simulink model "simulink_scenario_reader"  (R2022a)
settings: Solver=FixedStepAuto  StartTime=0.0  StopTime=10.0  RelTol=1e-3
model workspace (MAT data in the model file):
  firstWarning = 0
  originalScenarioChecksum = 'E48F73370D4002DBAA47AD0521C44C41'
undefined symbols (not defined in the file or in its folder): driving
libraries: drivingscenarioandsensors x6, sim3dautolib x2, trackingutilitieslib x1, sim3dlib x1
settings Model: Creator=bighsiao  LastModifiedBy=bighsiao

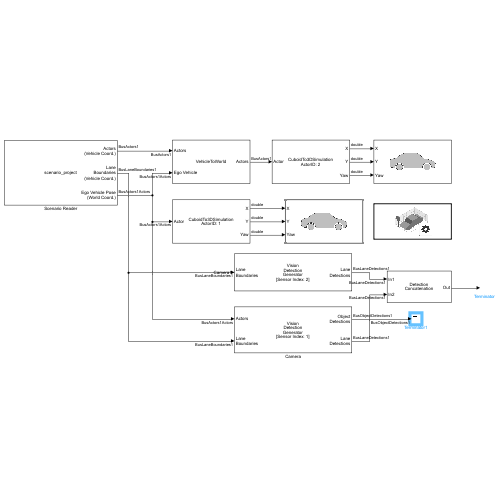
[thumbnail: Simulink's stored preview of the top-level diagram]
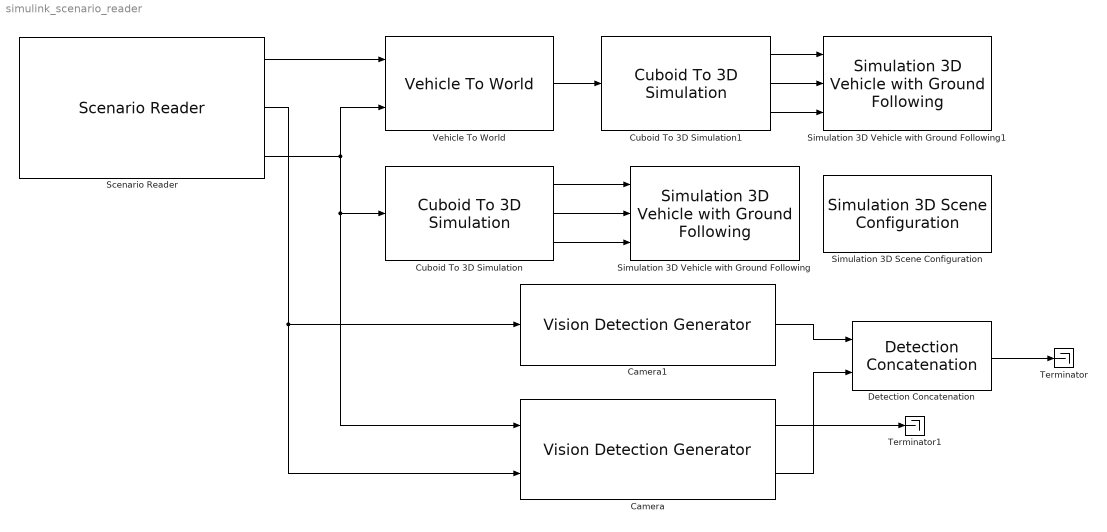
== system simulink_scenario_reader ==
  Camera : drivingscenarioandsensors/Vision Detection Generator  SensorIndex=1  DetectorOutput=Lanes and objects  UpdateInterval=0.1  LaneUpdateInterval=0.1  SensorLocation=[1.9 0]  Height=1.1  Yaw=0  Pitch=1  Roll=0  BusNameSource=Auto  BusName=BusObjectDetections  BusName2Source=Auto  BusName2=BusLaneDetections  MaxNumDetectionsSource=Property  MaxNumDetections=50  MaxNumLanesSource=Property  MaxNumLanes=30  DetectionCoordinates=Ego Cartesian  SimulateUsing=Interpreted execution  MaxRange=100  BoundingBoxAccuracy=5  ProcessNoiseIntensity=5  MaxSpeed=100  MaxAllowedOcclusion=0.5  MinObjectImageSize=[15 15]  DetectionProbability=0.9  FalsePositivesPerImage=0.1  MinLaneImageSize=[20 3]  LaneBoundaryAccuracy=3  HasNoise=on  InitialSeedSource=Repeatable  InitialSeed=0  UsedSeed=0  ActorProfilesSource=From Scenario Reader block  ActorProfilesParameters=driving.internal.ActorProfilesParameters  ActorProfilesExpression=[struct('ActorID',1,'ClassID',1,'Length',4.7,'Width',1.8,'Height',1.4,'OriginOffset',[-1.35 0 0],'MeshVertices',[3.7 0.9 0.857439446366782;3.7 -0.9 0.857439446366782;3.7 -0.9 0.314878892733564;3.7 0.9 0.314878892733564;3.7 0.9 0.857439446366782;2.525 0.9 0.993079584775086;2.525 -0.9 0.993079584775086;3.7 -0.9 0.857439446366782;1.82 0.72 1.4;0.41 0.72 1.4;0.41 -0.72 1.4;1.82 -0.72 1.4;-0.295 0.9 0.993079584775086;-1 0.9 0.857439446366782;-1 -0.9 0.857439446366782;-0.295 -0.9 0.993079584775086;3.7 0.9 0.857439446366782;3.7 0.9 0.314878892733564;2.525 0.9 0.314878892733564;2.525 0.9 0.993079584775086;2.525 0.9 0.993079584775086;2.525 0.9 0.314878892733564;-0.295 0.9 0.314878892733564;-0.295 0.9 0.993079584775086;-0.295 0.9 0.993079584775086;-0.295 0.9 0.314878892733564;-1 0.9 0.355570934256055;-1 0.9 0.857439446366782;2.525 0.9 0.993079584775086;-0.295 0.9 0.993079584775086;0.41 0.72 1.4;1.82 0.72 1.4;3.7 -0.9 0.857439446366782;3.7 -0.9 0.314878892733564;2.525 -0.9 0.314878892733564;2.525 -0.9 0.993079584775086;2.525 -0.9 0.993079584775086;2.525 -0.9 0.314878892733564;-0.295 -0.9 0.314878892733564;-0.295 -0.9 0.993079584775086;-0.295 -0.9 0.993079584775086;-0.295 -0.9 0.314878892733564;-1 -0.9 0.355570934256055;-1 -0.9 0.857439446366782;2.525 -0.9 0.993079584775086;-0.295 -0.9 0.993079584775086;0.41 -0.72 1.4;1.82 -0.72 1.4;-0.295 0.9 0.993079584775086;-0.295 -0.9 0.993079584775086;0.41 -0.72 1.4;0.41 0.72 1.4;2.525 -0.9 0.993079584775086;1.82 -0.72 1.4;1.82 0.72 1.4;2.525 0.9 0.993079584775086;-1 0.9 0.857439446366782;-1 0.9 0.355570934256055;-1 -0.9 0.355570934256055;-1 -0.9 0.857439446366782;3.7 0.9 0.314878892733564;3.7 -0.9 0.314878892733564;-0.295 -0.9 0.314878892733564;-0.295 0.9 0.314878892733564;-0.295 0.9 0.314878892733564;-1 0.9 0.355570934256055;-1 -0.9 0.355570934256055;-0.295 -0.9 0.314878892733564;0 -0.63 0;0 -0.87 0;0.191030206995054 -0.63 0.0601365173421445;0.191030206995054 -0.87 0.0601365173421445;0.309093367795925 -0.63 0.217575963708927;0.309093367795925 -0.87 0.217575963708927;0.309093367795925 -0.63 0.412181821758201;0.309093367795925 -0.87 0.412181821758201;0.191030206995054 -0.63 0.569621268124983;0.191030206995054 -0.87 0.569621268124983;0 -0.63 0.629757785467128;0 -0.87 0.629757785467128;-0.191030206995054 -0.63 0.569621268124983;-0.191030206995054 -0.87 0.569621268124983;-0.309093367795925 -0.63 0.412181821758201;-0.309093367795925 -0.87 0.412181821758201;-0.309093367795925 -0.63 0.217575963708927;-0.309093367795925 -0.87 0.217575963708927;-0.191030206995054 -0.63 0.0601365173421445;-0.191030206995054 -0.87 0.0601365173421445;0 -0.63 0;0 -0.87 0;0 -0.63 0;0.191030206995054 -0.63 0.0601365173421445;0.309093367795925 -0.63 0.217575963708927;0.309093367795925 -0.63 0.412181821758201;0.191030206995054 -0.63 0.569621268124983;0 -0.63 0.629757785467128;-0.191030206995054 -0.63 0.569621268124983;-0.309093367795925 -0.63 0.412181821758201;-0.309093367795925 -0.63 0.217575963708927;-0.191030206995054 -0.63 0.0601365173421445;0 -0.87 0;0.191030206995054 -0.87 0.0601365173421445;0.309093367795925 -0.87 0.217575963708927;0.309093367795925 -0.87 0.412181821758201;0.191030206995054 -0.87 0.569621268124983;0 -0.87 0.629757785467128;-0.191030206995054 -0.87 0.569621268124983;-0.309093367795925 -0.87 0.412181821758201;-0.309093367795925 -0.87 0.217575963708927;-0.191030206995054 -0.87 0.0601365173421445;0 0.87 0;0 0.63 0;0.191030206995054 0.87 0.0601365173421445;0.191030206995054 0.63 0.0601365173421445;0.309093367795925 0.87 0.217575963708927;0.309093367795925 0.63 0.217575963708927;0.309093367795925 0.87 0.412181821758201;0.309093367795925 0.63 0.412181821758201;0.191030206995054 0.87 0.569621268124983;0.191030206995054 0.63 0.569621268124983;0 0.87 0.629757785467128;0 0.63 0.629757785467128;-0.191030206995054 0.87 0.569621268124983;-0.191030206995054 0.63 0.569621268124983;-0.309093367795925 0.87 0.412181821758201;-0.309093367795925 0.63 0.412181821758201;-0.309093367795925 0.87 0.217575963708927;-0.309093367795925 0.63 0.217575963708927;-0.191030206995054 0.87 0.0601365173421445;-0.191030206995054 0.63 0.0601365173421445;0 ...(+3718 chars)],'MeshFaces',[1 2 3;3 4 1;5 6 7;7 8 5;9 10 11;11 12 9;13 14 15;15 16 13;17 18 19;19 20 17;21 22 23;23 24 21;25 26 27;27 28 25;29 30 31;31 32 29;33 34 35;35 36 33;37 38 39;39 40 37;41 42 43;43 44 41;45 46 47;47 48 45;49 50 51;51 52 49;53 54 55;55 56 53;57 58 59;59 60 57;61 62 63;63 64 61;65 66 67;67 68 65;69 71 72;72 70 69;71 73 74;74 72 71;73 75 76;76 74 73;75 77 78;78 76 75;77 79 80;80 78 77;79 81 82;82 80 79;81 83 84;84 82 81;83 85 86;86 84 83;85 87 88;88 86 85;87 89 90;90 88 87;91 92 93;91 93 94;91 94 95;91 95 96;91 96 97;91 97 98;91 98 99;91 99 100;101 102 103;101 103 104;101 104 105;101 105 106;101 106 107;101 107 108;101 108 109;101 109 110;111 113 114;114 112 111;113 115 116;116 114 113;115 117 118;118 116 115;117 119 120;120 118 117;119 121 122;122 120 119;121 123 124;124 122 121;123 125 126;126 124 123;125 127 128;128 126 125;127 129 130;130 128 127;129 131 132;132 130 129;133 134 135;133 135 136;133 136 137;133 137 138;133 138 139;133 139 140;133 140 141;133 141 142;143 144 145;143 145 146;143 146 147;143 147 148;143 148 149;143 149 150;143 150 151;143 151 152;153 155 156;156 154 153;155 157 158;158 156 155;157 159 160;160 158 157;159 161 162;162 160 159;161 163 164;164 162 161;163 165 166;166 164 163;165 167 168;168 166 165;167 169 170;170 168 167;169 171 172;172 170 169;171 173 174;174 172 171;175 176 177;175 177 178;175 178 179;175 179 180;175 180 181;175 181 182;175 182 183;175 183 184;185 186 187;185 187 188;185 188 189;185 189 190;185 190 191;185 191 192;185 192 193;185 193 194;195 197 198;198 196 195;197 199 200;200 198 197;199 201 202;202 200 199;201 203 204;204 202 201;203 205 206;206 204 203;205 207 208;208 206 205;207 209 210;210 208 207;209 211 212;212 210 209;211 213 214;214 212 211;213 215 216;216 214 213;217 218 219;217 219 220;217 220 221;217 221 222;217 222 223;217 223 224;217 224 225;217 225 226;227 228 229;227 229 230;227 230 231;227 231 232;227 232 233;227 233 234;227 234 235;227 235 236],'RCSPattern',[10 10;10 10],'RCSAzimuthAngles',[-180 180],'RCSElevationAngles',[-90 90]); struct('ActorID',2,'ClassID',2,'Length',8.2,'Width',2.5,'Height',3.5,'OriginOffset',[-3.1 0 0],'MeshVertices',[7.2 1.25 1.30597014925373;7.2 -1.25 1.30597014925373;7.2 -1.25 0.574626865671641;7.2 1.25 0.574626865671641;7.2 1.25 1.30597014925373;5.765 1.25 1.67164179104478;5.765 -1.25 1.67164179104478;7.2 -1.25 1.30597014925373;4.945 1 2.58582089552239;4.002 1 2.58582089552239;4.002 -1 2.58582089552239;4.945 -1 2.58582089552239;4.002 1 2.58582089552239;4.002 1.25 1.67164179104478;4.002 -1.25 1.67164179104478;4.002 -1 2.58582089552239;4.002 1.25 1.67164179104478;4.002 1.25 0.574626865671641;4.002 -1.25 0.574626865671641;4.002 -1.25 1.67164179104478;3.92 1.25 3.5;-1 1.25 3.5;-1 -1.25 3.5;3.92 -1.25 3.5;3.92 -1.25 3.5;3.92 -1.25 0.574626865671641;3.92 1.25 0.574626865671641;3.92 1.25 3.5;-1 1.25 3.5;-1 1.25 0.574626865671641;3.92 1.25 0.574626865671641;3.92 1.25 3.5;-1 -1.25 3.5;-1 -1.25 0.574626865671641;3.92 -1.25 0.574626865671641;3.92 -1.25 3.5;5.765 1.25 1.67164179104478;5.355 1.25 1.67164179104478;4.74 1 2.58582089552239;4.945 1 2.58582089552239;7.2 1.25 1.30597014925373;7.2 1.25 0.574626865671641;5.765 1.25 0.574626865671641;5.765 1.25 1.67164179104478;5.765 1.25 1.67164179104478;5.765 1.25 0.574626865671641;4.002 1.25 0.574626865671641;4.002 1.25 1.67164179104478;4.33 1.25 1.67164179104478;4.002 1.25 1.67164179104478;4.002 1 2.58582089552239;4.33 1 2.58582089552239;5.765 -1.25 1.67164179104478;5.355 -1.25 1.67164179104478;4.74 -1 2.58582089552239;4.945 -1 2.58582089552239;7.2 -1.25 1.30597014925373;7.2 -1.25 0.574626865671641;5.765 -1.25 0.574626865671641;5.765 -1.25 1.67164179104478;5.765 -1.25 1.67164179104478;5.765 -1.25 0.574626865671641;4.002 -1.25 0.574626865671641;4.002 -1.25 1.67164179104478;4.33 -1.25 1.67164179104478;4.002 -1.25 1.67164179104478;4.002 -1 2.58582089552239;4.33 -1 2.58582089552239;-1 1.25 3.5;-1 1.25 0.574626865671641;-1 -1.25 0.574626865671641;-1 -1.25 3.5;7.2 1.25 0.574626865671641;7.2 -1.25 0.574626865671641;-1 -1.25 0.574626865671641;-1 1.25 0.574626865671641;0 -0.915 -2.22044604925031e-16;0 -1.185 -2.22044604925031e-16;0.293892626146237 -0.915 0.0997672417444302;0.293892626146237 -1.185 0.0997672417444302;0.475528258147577 -0.915 0.360961271595177;0.475528258147577 -1.185 0.360961271595177;0.475528258147577 -0.915 0.683814847807808;0.475528258147577 -1.185 0.683814847807808;0.293892626146237 -0.915 0.945008877658554;0.293892626146237 -1.185 0.945008877658554;0 -0.915 1.04477611940298;0 -1.185 1.04477611940298;-0.293892626146237 -0.915 0.945008877658554;-0.293892626146237 -1.185 0.945008877658554;-0.475528258147577 -0.915 0.683814847807808;-0.475528258147577 -1.185 0.683814847807808;-0.475528258147577 -0.915 0.360961271595177;-0.475528258147577 -1.185 0.360961271595177;-0.293892626146237 -0.915 0.0997672417444302;-0.293892626146237 -1.185 0.0997672417444302;0 -0.915 -2.22044604925031e-16;0 -1.185 -2.22044604925031e-16;0 -0.915 -2.22044604925031e-16;0.293892626146237 -0.915 0.0997672417444302;0.475528258147577 -0.915 0.360961271595177;0.475528258147577 -0.915 0.683814847807808;0.293892626146237 -0.915 0.945008877658554;0 -0.915 1.04477611940298;-0.293892626146237 -0.915 0.945008877658554;-0.475528258147577 -0.915 0.683814847807808;-0.475528258147577 -0.915 0.360961271595177;-0.293892626146237 -0.915 0.0997672417444302;0 -1.185 -2.22044604925031e-16;0.293892626146237 -1.185 0.0997672417444302;0.475528258147577 -1.185 0.360961271595177;0.475528258147577 -1.185 0.683814847807808;0.293892626146237 -1.185 0.945008877658554;0 -1.185 1.04477611940298;-0.293892626146237 -1.185 0.945008877658554;-0.475528258147577 -1.185 0.683814847807808;-0.475528258147577 -1.185 0.360961271595177;-0.293892626146237 -1.185 0.0997672417444302;0 1.185 -2.22044604925031e-16;0 0.915 -2.22044604925031e-16;0.293892626146237 1.185 0.0997672417444302;0.293892626146237 0.915 0.0997672417444302;0.475528258147577 1.185 0.360961271595177;0.475528258147577 0.915 0.360961271595177;0.475528258147577 1.185 0.683814847807808;0.475528258147577 0.915 0.683814847807808;0.293892626146237 1.185 0.945008877658554;0.293892626146237 0.915 ...(+7888 chars)],'MeshFaces',[1 2 3;3 4 1;5 6 7;7 8 5;9 10 11;11 12 9;13 14 15;15 16 13;17 18 19;19 20 17;21 22 23;23 24 21;25 26 27;27 28 25;29 30 31;31 32 29;33 34 35;35 36 33;37 38 39;39 40 37;41 42 43;43 44 41;45 46 47;47 48 45;49 50 51;51 52 49;53 54 55;55 56 53;57 58 59;59 60 57;61 62 63;63 64 61;65 66 67;67 68 65;69 70 71;71 72 69;73 74 75;75 76 73;77 79 80;80 78 77;79 81 82;82 80 79;81 83 84;84 82 81;83 85 86;86 84 83;85 87 88;88 86 85;87 89 90;90 88 87;89 91 92;92 90 89;91 93 94;94 92 91;93 95 96;96 94 93;95 97 98;98 96 95;99 100 101;99 101 102;99 102 103;99 103 104;99 104 105;99 105 106;99 106 107;99 107 108;109 110 111;109 111 112;109 112 113;109 113 114;109 114 115;109 115 116;109 116 117;109 117 118;119 121 122;122 120 119;121 123 124;124 122 121;123 125 126;126 124 123;125 127 128;128 126 125;127 129 130;130 128 127;129 131 132;132 130 129;131 133 134;134 132 131;133 135 136;136 134 133;135 137 138;138 136 135;137 139 140;140 138 137;141 142 143;141 143 144;141 144 145;141 145 146;141 146 147;141 147 148;141 148 149;141 149 150;151 152 153;151 153 154;151 154 155;151 155 156;151 156 157;151 157 158;151 158 159;151 159 160;161 163 164;164 162 161;163 165 166;166 164 163;165 167 168;168 166 165;167 169 170;170 168 167;169 171 172;172 170 169;171 173 174;174 172 171;173 175 176;176 174 173;175 177 178;178 176 175;177 179 180;180 178 177;179 181 182;182 180 179;183 184 185;183 185 186;183 186 187;183 187 188;183 188 189;183 189 190;183 190 191;183 191 192;193 194 195;193 195 196;193 196 197;193 197 198;193 198 199;193 199 200;193 200 201;193 201 202;203 205 206;206 204 203;205 207 208;208 206 205;207 209 210;210 208 207;209 211 212;212 210 209;211 213 214;214 212 211;213 215 216;216 214 213;215 217 218;218 216 215;217 219 220;220 218 217;219 221 222;222 220 219;221 223 224;224 222 221;225 226 227;225 227 228;225 228 229;225 229 230;225 230 231;225 231 232;225 232 233;225 233 234;235 236 237;235 237 238;235 238 239;235 239 240;235 240 241;235 241 242;235 242 243;235 243 244;245 247 248;248 246 245;247 249 250;250 248 247;249 251 252;252 250 249;251 253 254;254 252 251;253 255 256;256 254 253;255 257 258;258 256 255;257 259 260;260 258 257;259 261 262;262 260 259;261 263 264;264 262 261;263 265 266;266 264 263;267 268 269;267 269 270;267 270 271;267 271 272;267 272 273;267 273 274;267 274 275;267 275 276;277 278 279;277 279 280;277 280 281;277 281 282;277 282 283;277 283 284;277 284 285;277 285 286;287 289 290;290 288 287;289 291 292;292 290 289;291 293 294;294 292 291;293 295 296;296 294 293;295 297 298;298 296 295;297 299 300;300 298 297;299 301 302;302 300 299;301 303 304;304 302 301;303 305 306;306 304 303;305 307 308;308 306 305;309 310 311;309 311 312;309 312 313;309 313 314;309 314 315;309 315 316;309 316 317;309 317 318;319 320 321;319 321 322;319 322 323;319 323 324;319 324 325;319 325 326;319 326 327;319 327 328],'RCSPattern',[10 10;10 10],'RCSAzimuthAngles',[-180 180],'RCSElevationAngles',[-90 90])]  Intrinsics=driving.internal.cameraIntrinsics('FocalLength',[500 1814.81],'PrincipalPoint',[320 240],'ImageSize',[720 480],'RadialDistortion',[0 0],'TangentialDistortion',[0 0],'Skew',0)
  Camera1 : drivingscenarioandsensors/Vision Detection Generator  SensorIndex=2  DetectorOutput=Lanes only  UpdateInterval=0.1  LaneUpdateInterval=0.1  SensorLocation=[-1 0]  Height=1.1  Yaw=-180  Pitch=1  Roll=0  BusNameSource=Auto  BusName=BusObjectDetections  BusName2Source=Auto  BusName2=BusLaneDetections  MaxNumDetectionsSource=Property  MaxNumDetections=50  MaxNumLanesSource=Property  MaxNumLanes=30  DetectionCoordinates=Ego Cartesian  SimulateUsing=Interpreted execution  MaxRange=150  BoundingBoxAccuracy=5  ProcessNoiseIntensity=5  MaxSpeed=100  MaxAllowedOcclusion=0.5  MinObjectImageSize=[15 15]  DetectionProbability=0.9  FalsePositivesPerImage=0.1  MinLaneImageSize=[20 3]  LaneBoundaryAccuracy=3  HasNoise=on  InitialSeedSource=Repeatable  InitialSeed=0  UsedSeed=0  ActorProfilesSource=From Scenario Reader block  ActorProfilesParameters=driving.internal.ActorProfilesParameters  ActorProfilesExpression=[struct('ActorID',1,'ClassID',1,'Length',4.7,'Width',1.8,'Height',1.4,'OriginOffset',[-1.35 0 0],'MeshVertices',[3.7 0.9 0.857439446366782;3.7 -0.9 0.857439446366782;3.7 -0.9 0.314878892733564;3.7 0.9 0.314878892733564;3.7 0.9 0.857439446366782;2.525 0.9 0.993079584775086;2.525 -0.9 0.993079584775086;3.7 -0.9 0.857439446366782;1.82 0.72 1.4;0.41 0.72 1.4;0.41 -0.72 1.4;1.82 -0.72 1.4;-0.295 0.9 0.993079584775086;-1 0.9 0.857439446366782;-1 -0.9 0.857439446366782;-0.295 -0.9 0.993079584775086;3.7 0.9 0.857439446366782;3.7 0.9 0.314878892733564;2.525 0.9 0.314878892733564;2.525 0.9 0.993079584775086;2.525 0.9 0.993079584775086;2.525 0.9 0.314878892733564;-0.295 0.9 0.314878892733564;-0.295 0.9 0.993079584775086;-0.295 0.9 0.993079584775086;-0.295 0.9 0.314878892733564;-1 0.9 0.355570934256055;-1 0.9 0.857439446366782;2.525 0.9 0.993079584775086;-0.295 0.9 0.993079584775086;0.41 0.72 1.4;1.82 0.72 1.4;3.7 -0.9 0.857439446366782;3.7 -0.9 0.314878892733564;2.525 -0.9 0.314878892733564;2.525 -0.9 0.993079584775086;2.525 -0.9 0.993079584775086;2.525 -0.9 0.314878892733564;-0.295 -0.9 0.314878892733564;-0.295 -0.9 0.993079584775086;-0.295 -0.9 0.993079584775086;-0.295 -0.9 0.314878892733564;-1 -0.9 0.355570934256055;-1 -0.9 0.857439446366782;2.525 -0.9 0.993079584775086;-0.295 -0.9 0.993079584775086;0.41 -0.72 1.4;1.82 -0.72 1.4;-0.295 0.9 0.993079584775086;-0.295 -0.9 0.993079584775086;0.41 -0.72 1.4;0.41 0.72 1.4;2.525 -0.9 0.993079584775086;1.82 -0.72 1.4;1.82 0.72 1.4;2.525 0.9 0.993079584775086;-1 0.9 0.857439446366782;-1 0.9 0.355570934256055;-1 -0.9 0.355570934256055;-1 -0.9 0.857439446366782;3.7 0.9 0.314878892733564;3.7 -0.9 0.314878892733564;-0.295 -0.9 0.314878892733564;-0.295 0.9 0.314878892733564;-0.295 0.9 0.314878892733564;-1 0.9 0.355570934256055;-1 -0.9 0.355570934256055;-0.295 -0.9 0.314878892733564;0 -0.63 0;0 -0.87 0;0.191030206995054 -0.63 0.0601365173421445;0.191030206995054 -0.87 0.0601365173421445;0.309093367795925 -0.63 0.217575963708927;0.309093367795925 -0.87 0.217575963708927;0.309093367795925 -0.63 0.412181821758201;0.309093367795925 -0.87 0.412181821758201;0.191030206995054 -0.63 0.569621268124983;0.191030206995054 -0.87 0.569621268124983;0 -0.63 0.629757785467128;0 -0.87 0.629757785467128;-0.191030206995054 -0.63 0.569621268124983;-0.191030206995054 -0.87 0.569621268124983;-0.309093367795925 -0.63 0.412181821758201;-0.309093367795925 -0.87 0.412181821758201;-0.309093367795925 -0.63 0.217575963708927;-0.309093367795925 -0.87 0.217575963708927;-0.191030206995054 -0.63 0.0601365173421445;-0.191030206995054 -0.87 0.0601365173421445;0 -0.63 0;0 -0.87 0;0 -0.63 0;0.191030206995054 -0.63 0.0601365173421445;0.309093367795925 -0.63 0.217575963708927;0.309093367795925 -0.63 0.412181821758201;0.191030206995054 -0.63 0.569621268124983;0 -0.63 0.629757785467128;-0.191030206995054 -0.63 0.569621268124983;-0.309093367795925 -0.63 0.412181821758201;-0.309093367795925 -0.63 0.217575963708927;-0.191030206995054 -0.63 0.0601365173421445;0 -0.87 0;0.191030206995054 -0.87 0.0601365173421445;0.309093367795925 -0.87 0.217575963708927;0.309093367795925 -0.87 0.412181821758201;0.191030206995054 -0.87 0.569621268124983;0 -0.87 0.629757785467128;-0.191030206995054 -0.87 0.569621268124983;-0.309093367795925 -0.87 0.412181821758201;-0.309093367795925 -0.87 0.217575963708927;-0.191030206995054 -0.87 0.0601365173421445;0 0.87 0;0 0.63 0;0.191030206995054 0.87 0.0601365173421445;0.191030206995054 0.63 0.0601365173421445;0.309093367795925 0.87 0.217575963708927;0.309093367795925 0.63 0.217575963708927;0.309093367795925 0.87 0.412181821758201;0.309093367795925 0.63 0.412181821758201;0.191030206995054 0.87 0.569621268124983;0.191030206995054 0.63 0.569621268124983;0 0.87 0.629757785467128;0 0.63 0.629757785467128;-0.191030206995054 0.87 0.569621268124983;-0.191030206995054 0.63 0.569621268124983;-0.309093367795925 0.87 0.412181821758201;-0.309093367795925 0.63 0.412181821758201;-0.309093367795925 0.87 0.217575963708927;-0.309093367795925 0.63 0.217575963708927;-0.191030206995054 0.87 0.0601365173421445;-0.191030206995054 0.63 0.0601365173421445;0 ...(+3718 chars)],'MeshFaces',[1 2 3;3 4 1;5 6 7;7 8 5;9 10 11;11 12 9;13 14 15;15 16 13;17 18 19;19 20 17;21 22 23;23 24 21;25 26 27;27 28 25;29 30 31;31 32 29;33 34 35;35 36 33;37 38 39;39 40 37;41 42 43;43 44 41;45 46 47;47 48 45;49 50 51;51 52 49;53 54 55;55 56 53;57 58 59;59 60 57;61 62 63;63 64 61;65 66 67;67 68 65;69 71 72;72 70 69;71 73 74;74 72 71;73 75 76;76 74 73;75 77 78;78 76 75;77 79 80;80 78 77;79 81 82;82 80 79;81 83 84;84 82 81;83 85 86;86 84 83;85 87 88;88 86 85;87 89 90;90 88 87;91 92 93;91 93 94;91 94 95;91 95 96;91 96 97;91 97 98;91 98 99;91 99 100;101 102 103;101 103 104;101 104 105;101 105 106;101 106 107;101 107 108;101 108 109;101 109 110;111 113 114;114 112 111;113 115 116;116 114 113;115 117 118;118 116 115;117 119 120;120 118 117;119 121 122;122 120 119;121 123 124;124 122 121;123 125 126;126 124 123;125 127 128;128 126 125;127 129 130;130 128 127;129 131 132;132 130 129;133 134 135;133 135 136;133 136 137;133 137 138;133 138 139;133 139 140;133 140 141;133 141 142;143 144 145;143 145 146;143 146 147;143 147 148;143 148 149;143 149 150;143 150 151;143 151 152;153 155 156;156 154 153;155 157 158;158 156 155;157 159 160;160 158 157;159 161 162;162 160 159;161 163 164;164 162 161;163 165 166;166 164 163;165 167 168;168 166 165;167 169 170;170 168 167;169 171 172;172 170 169;171 173 174;174 172 171;175 176 177;175 177 178;175 178 179;175 179 180;175 180 181;175 181 182;175 182 183;175 183 184;185 186 187;185 187 188;185 188 189;185 189 190;185 190 191;185 191 192;185 192 193;185 193 194;195 197 198;198 196 195;197 199 200;200 198 197;199 201 202;202 200 199;201 203 204;204 202 201;203 205 206;206 204 203;205 207 208;208 206 205;207 209 210;210 208 207;209 211 212;212 210 209;211 213 214;214 212 211;213 215 216;216 214 213;217 218 219;217 219 220;217 220 221;217 221 222;217 222 223;217 223 224;217 224 225;217 225 226;227 228 229;227 229 230;227 230 231;227 231 232;227 232 233;227 233 234;227 234 235;227 235 236],'RCSPattern',[10 10;10 10],'RCSAzimuthAngles',[-180 180],'RCSElevationAngles',[-90 90]); struct('ActorID',2,'ClassID',2,'Length',8.2,'Width',2.5,'Height',3.5,'OriginOffset',[-3.1 0 0],'MeshVertices',[7.2 1.25 1.30597014925373;7.2 -1.25 1.30597014925373;7.2 -1.25 0.574626865671641;7.2 1.25 0.574626865671641;7.2 1.25 1.30597014925373;5.765 1.25 1.67164179104478;5.765 -1.25 1.67164179104478;7.2 -1.25 1.30597014925373;4.945 1 2.58582089552239;4.002 1 2.58582089552239;4.002 -1 2.58582089552239;4.945 -1 2.58582089552239;4.002 1 2.58582089552239;4.002 1.25 1.67164179104478;4.002 -1.25 1.67164179104478;4.002 -1 2.58582089552239;4.002 1.25 1.67164179104478;4.002 1.25 0.574626865671641;4.002 -1.25 0.574626865671641;4.002 -1.25 1.67164179104478;3.92 1.25 3.5;-1 1.25 3.5;-1 -1.25 3.5;3.92 -1.25 3.5;3.92 -1.25 3.5;3.92 -1.25 0.574626865671641;3.92 1.25 0.574626865671641;3.92 1.25 3.5;-1 1.25 3.5;-1 1.25 0.574626865671641;3.92 1.25 0.574626865671641;3.92 1.25 3.5;-1 -1.25 3.5;-1 -1.25 0.574626865671641;3.92 -1.25 0.574626865671641;3.92 -1.25 3.5;5.765 1.25 1.67164179104478;5.355 1.25 1.67164179104478;4.74 1 2.58582089552239;4.945 1 2.58582089552239;7.2 1.25 1.30597014925373;7.2 1.25 0.574626865671641;5.765 1.25 0.574626865671641;5.765 1.25 1.67164179104478;5.765 1.25 1.67164179104478;5.765 1.25 0.574626865671641;4.002 1.25 0.574626865671641;4.002 1.25 1.67164179104478;4.33 1.25 1.67164179104478;4.002 1.25 1.67164179104478;4.002 1 2.58582089552239;4.33 1 2.58582089552239;5.765 -1.25 1.67164179104478;5.355 -1.25 1.67164179104478;4.74 -1 2.58582089552239;4.945 -1 2.58582089552239;7.2 -1.25 1.30597014925373;7.2 -1.25 0.574626865671641;5.765 -1.25 0.574626865671641;5.765 -1.25 1.67164179104478;5.765 -1.25 1.67164179104478;5.765 -1.25 0.574626865671641;4.002 -1.25 0.574626865671641;4.002 -1.25 1.67164179104478;4.33 -1.25 1.67164179104478;4.002 -1.25 1.67164179104478;4.002 -1 2.58582089552239;4.33 -1 2.58582089552239;-1 1.25 3.5;-1 1.25 0.574626865671641;-1 -1.25 0.574626865671641;-1 -1.25 3.5;7.2 1.25 0.574626865671641;7.2 -1.25 0.574626865671641;-1 -1.25 0.574626865671641;-1 1.25 0.574626865671641;0 -0.915 -2.22044604925031e-16;0 -1.185 -2.22044604925031e-16;0.293892626146237 -0.915 0.0997672417444302;0.293892626146237 -1.185 0.0997672417444302;0.475528258147577 -0.915 0.360961271595177;0.475528258147577 -1.185 0.360961271595177;0.475528258147577 -0.915 0.683814847807808;0.475528258147577 -1.185 0.683814847807808;0.293892626146237 -0.915 0.945008877658554;0.293892626146237 -1.185 0.945008877658554;0 -0.915 1.04477611940298;0 -1.185 1.04477611940298;-0.293892626146237 -0.915 0.945008877658554;-0.293892626146237 -1.185 0.945008877658554;-0.475528258147577 -0.915 0.683814847807808;-0.475528258147577 -1.185 0.683814847807808;-0.475528258147577 -0.915 0.360961271595177;-0.475528258147577 -1.185 0.360961271595177;-0.293892626146237 -0.915 0.0997672417444302;-0.293892626146237 -1.185 0.0997672417444302;0 -0.915 -2.22044604925031e-16;0 -1.185 -2.22044604925031e-16;0 -0.915 -2.22044604925031e-16;0.293892626146237 -0.915 0.0997672417444302;0.475528258147577 -0.915 0.360961271595177;0.475528258147577 -0.915 0.683814847807808;0.293892626146237 -0.915 0.945008877658554;0 -0.915 1.04477611940298;-0.293892626146237 -0.915 0.945008877658554;-0.475528258147577 -0.915 0.683814847807808;-0.475528258147577 -0.915 0.360961271595177;-0.293892626146237 -0.915 0.0997672417444302;0 -1.185 -2.22044604925031e-16;0.293892626146237 -1.185 0.0997672417444302;0.475528258147577 -1.185 0.360961271595177;0.475528258147577 -1.185 0.683814847807808;0.293892626146237 -1.185 0.945008877658554;0 -1.185 1.04477611940298;-0.293892626146237 -1.185 0.945008877658554;-0.475528258147577 -1.185 0.683814847807808;-0.475528258147577 -1.185 0.360961271595177;-0.293892626146237 -1.185 0.0997672417444302;0 1.185 -2.22044604925031e-16;0 0.915 -2.22044604925031e-16;0.293892626146237 1.185 0.0997672417444302;0.293892626146237 0.915 0.0997672417444302;0.475528258147577 1.185 0.360961271595177;0.475528258147577 0.915 0.360961271595177;0.475528258147577 1.185 0.683814847807808;0.475528258147577 0.915 0.683814847807808;0.293892626146237 1.185 0.945008877658554;0.293892626146237 0.915 ...(+7888 chars)],'MeshFaces',[1 2 3;3 4 1;5 6 7;7 8 5;9 10 11;11 12 9;13 14 15;15 16 13;17 18 19;19 20 17;21 22 23;23 24 21;25 26 27;27 28 25;29 30 31;31 32 29;33 34 35;35 36 33;37 38 39;39 40 37;41 42 43;43 44 41;45 46 47;47 48 45;49 50 51;51 52 49;53 54 55;55 56 53;57 58 59;59 60 57;61 62 63;63 64 61;65 66 67;67 68 65;69 70 71;71 72 69;73 74 75;75 76 73;77 79 80;80 78 77;79 81 82;82 80 79;81 83 84;84 82 81;83 85 86;86 84 83;85 87 88;88 86 85;87 89 90;90 88 87;89 91 92;92 90 89;91 93 94;94 92 91;93 95 96;96 94 93;95 97 98;98 96 95;99 100 101;99 101 102;99 102 103;99 103 104;99 104 105;99 105 106;99 106 107;99 107 108;109 110 111;109 111 112;109 112 113;109 113 114;109 114 115;109 115 116;109 116 117;109 117 118;119 121 122;122 120 119;121 123 124;124 122 121;123 125 126;126 124 123;125 127 128;128 126 125;127 129 130;130 128 127;129 131 132;132 130 129;131 133 134;134 132 131;133 135 136;136 134 133;135 137 138;138 136 135;137 139 140;140 138 137;141 142 143;141 143 144;141 144 145;141 145 146;141 146 147;141 147 148;141 148 149;141 149 150;151 152 153;151 153 154;151 154 155;151 155 156;151 156 157;151 157 158;151 158 159;151 159 160;161 163 164;164 162 161;163 165 166;166 164 163;165 167 168;168 166 165;167 169 170;170 168 167;169 171 172;172 170 169;171 173 174;174 172 171;173 175 176;176 174 173;175 177 178;178 176 175;177 179 180;180 178 177;179 181 182;182 180 179;183 184 185;183 185 186;183 186 187;183 187 188;183 188 189;183 189 190;183 190 191;183 191 192;193 194 195;193 195 196;193 196 197;193 197 198;193 198 199;193 199 200;193 200 201;193 201 202;203 205 206;206 204 203;205 207 208;208 206 205;207 209 210;210 208 207;209 211 212;212 210 209;211 213 214;214 212 211;213 215 216;216 214 213;215 217 218;218 216 215;217 219 220;220 218 217;219 221 222;222 220 219;221 223 224;224 222 221;225 226 227;225 227 228;225 228 229;225 229 230;225 230 231;225 231 232;225 232 233;225 233 234;235 236 237;235 237 238;235 238 239;235 239 240;235 240 241;235 241 242;235 242 243;235 243 244;245 247 248;248 246 245;247 249 250;250 248 247;249 251 252;252 250 249;251 253 254;254 252 251;253 255 256;256 254 253;255 257 258;258 256 255;257 259 260;260 258 257;259 261 262;262 260 259;261 263 264;264 262 261;263 265 266;266 264 263;267 268 269;267 269 270;267 270 271;267 271 272;267 272 273;267 273 274;267 274 275;267 275 276;277 278 279;277 279 280;277 280 281;277 281 282;277 282 283;277 283 284;277 284 285;277 285 286;287 289 290;290 288 287;289 291 292;292 290 289;291 293 294;294 292 291;293 295 296;296 294 293;295 297 298;298 296 295;297 299 300;300 298 297;299 301 302;302 300 299;301 303 304;304 302 301;303 305 306;306 304 303;305 307 308;308 306 305;309 310 311;309 311 312;309 312 313;309 313 314;309 314 315;309 315 316;309 316 317;309 317 318;319 320 321;319 321 322;319 322 323;319 323 324;319 324 325;319 325 326;319 326 327;319 327 328],'RCSPattern',[10 10;10 10],'RCSAzimuthAngles',[-180 180],'RCSElevationAngles',[-90 90])]  Intrinsics=driving.internal.cameraIntrinsics('FocalLength',[500 500],'PrincipalPoint',[320 240],'ImageSize',[720 480],'RadialDistortion',[0 0],'TangentialDistortion',[0 0],'Skew',0)
  Cuboid To 3D Simulation : drivingscenarioandsensors/Cuboid To 3D Simulation  SpecifyActorID=on  ActorIDToConvert=1  SimulateUsing=Interpreted execution
      settings: SourceProductBaseCode=DR
  Cuboid To 3D Simulation1 : drivingscenarioandsensors/Cuboid To 3D Simulation  SpecifyActorID=on  ActorIDToConvert=2  SimulateUsing=Interpreted execution
      settings: SourceProductBaseCode=DR
  Detection Concatenation : trackingutilitieslib/Detection Concatenation  NumInputs=2  BusNameSource=Auto  BusName=BusDetectionConcatenation  SimulateUsing=Interpreted execution
      settings: SourceProductBaseCode=TF,AE,DR,RA,UV,VE
  Scenario Reader : drivingscenarioandsensors/Scenario Reader  ScenarioSource=From file  ScenarioFileName=C:\Users\bighsiao\Desktop\matlab_project\scenario_project.mat  ScenarioVariableName=scenario  OutputCoordinateSystem=Vehicle coordinates  EgoVehicleSource=Scenario  EgoVehicleActorID=1  OrientVehiclesOnRoad=off  OutputEgoVehiclePose=on  OutputEgoVehicleState=off  SampleTime=0.1  LaneBoundaryOutput=Ego vehicle lane boundaries  LaneBoundaryDistance=0:0.5:9.5  LaneBoundaryLocation=Center of lane markings  BusNameSource=Auto  BusName=BusActors  BusNumActorsSource=Scenario  BusNumActors=100  BusName2Source=Auto  BusName2=BusLaneBoundaries  BusNumLaneBoundariesSource=Scenario  BusNumLaneBoundaries=10  BusName3Source=Auto  BusName3=BusEgoActor  BusName4Source=Auto  BusName4=BusEgoState  ShowCoordinateLabels=on  SimulateUsing=Interpreted execution
  Simulation 3D Scene Configuration : sim3dlib/Simulation 3D Scene Configuration  Priority=0  ProjectFormat=Default Scenes  SceneDesc=Straight road  ProjectName=C:\Program Files\MATLAB\R2022a\toolbox\shared\sim3d_projects\automotive_project\UE4\WindowsNoEditor\VehicleSimulation.exe  ScenePath=/Game/Maps/HwStrght  vehTagList={'Scene Origin';'SimulinkVehicle1';'SimulinkVehicle2'}  vehTag=Scene Origin  OpVisEn=off  Ts=1/60  EnableWindow=on  EnableRemoteAccess=off  EnableWeather=off  SunAltitude=40.0  SunAzimuth=90  clouds=10  wind=1  fog=0  rain=0  sensorTag=MainCamera1  sensorId=1  sensorName=MainCamera1  mountLoc=Origin  offsetFlag=off  tmountOffset=[0, 0, 0]  rmountOffset=[0, 0, 0]  HorizontalResolution=1280  VerticalResolution=720  HorizontalFOV=60  mountPoint=[0 0 0]  mountOrientation=[0 0 0]  aMode=3  ID=1
      settings: SourceProductBaseCode=VE,AE,DR,UV,VE
  Simulation 3D Vehicle with Ground Following : sim3dautolib/Simulation 3D Vehicle with Ground Following  Priority=-1  PassVehMesh=Muscle car  MeshPath=/MathWorksSimulation/Vehicles/Muscle/Meshes/SK_MuscleCar.SK_MuscleCar  TrackWidth=1.9  WheelBase=3  WheelRadius=0.35  VehColor=Red  InitialPos=[0, 0, 0]  InitialRot=[0, 0, 0]  ActorName=SimulinkVehicle1  SampleTime=-1  ActorType=SimulinkVehicle  ID=1  aMode=3  ActorTag=SimulinkVehicle1  CoordinateScheme=ISO  VehLightsControl=off  HeadlightColor=[ 1, 1, 1 ]  HighBeamIntensity=100000  LowBeamIntensity=60000  HighBeamConeAngle=70  LowBeamConeAngle=70  LeftHeadlightOrientation=[ 0, 0 ]  RightHeadlightOrientation=[ 0, 0 ]  BrakelightIntensity=500  ReverselightIntensity=500  SignallightIntensity=500  SignallightPeriod=1  SignalPulseWidth=50  TransformOutportEnabled=off
      settings: SourceProductBaseCode=VE,AE,DR,UV,VE
  Simulation 3D Vehicle with Ground Following1 : sim3dautolib/Simulation 3D Vehicle with Ground Following  Priority=-1  PassVehMesh=Box truck  MeshPath=/MathWorksSimulation/Vehicles/Muscle/Meshes/SK_MuscleCar.SK_MuscleCar  TrackWidth=1.9  WheelBase=3  WheelRadius=0.35  VehColor=Yellow  InitialPos=[0, 0, 0]  InitialRot=[0, 0, 0]  ActorName=SimulinkVehicle2  SampleTime=-1  ActorType=SimulinkVehicle  ID=2  aMode=3  ActorTag=SimulinkVehicle2  CoordinateScheme=ISO  VehLightsControl=off  HeadlightColor=[ 1, 1, 1 ]  HighBeamIntensity=100000  LowBeamIntensity=60000  HighBeamConeAngle=70  LowBeamConeAngle=70  LeftHeadlightOrientation=[ 0, 0 ]  RightHeadlightOrientation=[ 0, 0 ]  BrakelightIntensity=500  ReverselightIntensity=500  SignallightIntensity=500  SignallightPeriod=1  SignalPulseWidth=50  TransformOutportEnabled=off
      settings: SourceProductBaseCode=VE,AE,DR,UV,VE
  Terminator : Terminator
  Terminator1 : Terminator
  Vehicle To World : drivingscenarioandsensors/Vehicle To World  BusNameSource=Auto  BusName=BusVehicleToWorldActors  SimulateUsing=Interpreted execution
      settings: SourceProductBaseCode=DR
  wires:
  Vehicle To World/1 -> Cuboid To 3D Simulation1/1
  Cuboid To 3D Simulation1/1 -> Simulation 3D Vehicle with Ground Following1/1
  Scenario Reader/1 -> Vehicle To World/1
  Cuboid To 3D Simulation1/2 -> Simulation 3D Vehicle with Ground Following1/2
  Cuboid To 3D Simulation1/3 -> Simulation 3D Vehicle with Ground Following1/3
  Cuboid To 3D Simulation/2 -> Simulation 3D Vehicle with Ground Following/2
  Cuboid To 3D Simulation/1 -> Simulation 3D Vehicle with Ground Following/1
  Cuboid To 3D Simulation/3 -> Simulation 3D Vehicle with Ground Following/3
  Scenario Reader/3 -> Cuboid To 3D Simulation/1, Camera/1, Vehicle To World/2
  Scenario Reader/2 -> Camera1/1, Camera/2
  Detection Concatenation/1 -> Terminator/1
  Camera1/1 -> Detection Concatenation/1
  Camera/2 -> Detection Concatenation/2
  Camera/1 -> Terminator1/1
